simulink model "edda-ctc"  (R2021a)
settings: Solver=ode45  StartTime=0.0  StopTime=100  RelTol=1e-10
values from neighbouring files (symbols this model uses):
  g = 9.81    [alg1.m]    (also in alg2.m; edda-ctc-script.m; edda-pd-script.m)
  K0 = 1    [alg1.m]    (also in alg2.m = 10; edda-ctc-script.m = 10; edda-pd-script.m)
  K1 = 1    [alg1.m]    (also in alg2.m; edda-ctc-script.m; edda-pd-script.m)
  Theta1 = 3.1    [alg1.m]    (also in alg2.m; edda-ctc-script.m; edda-pd-script.m)
  Theta2 = 9.5    [alg1.m]    (also in alg2.m; edda-ctc-script.m; edda-pd-script.m)
  Theta3 = 0.24    [alg1.m]    (also in alg2.m; edda-ctc-script.m; edda-pd-script.m)
  Theta4 = 0.77    [alg1.m]    (also in alg2.m; edda-ctc-script.m; edda-pd-script.m)
settings Model: Creator=lajk0  LastModifiedBy=lajk0
settings DataIOCC: ReturnWorkspaceOutputs=off

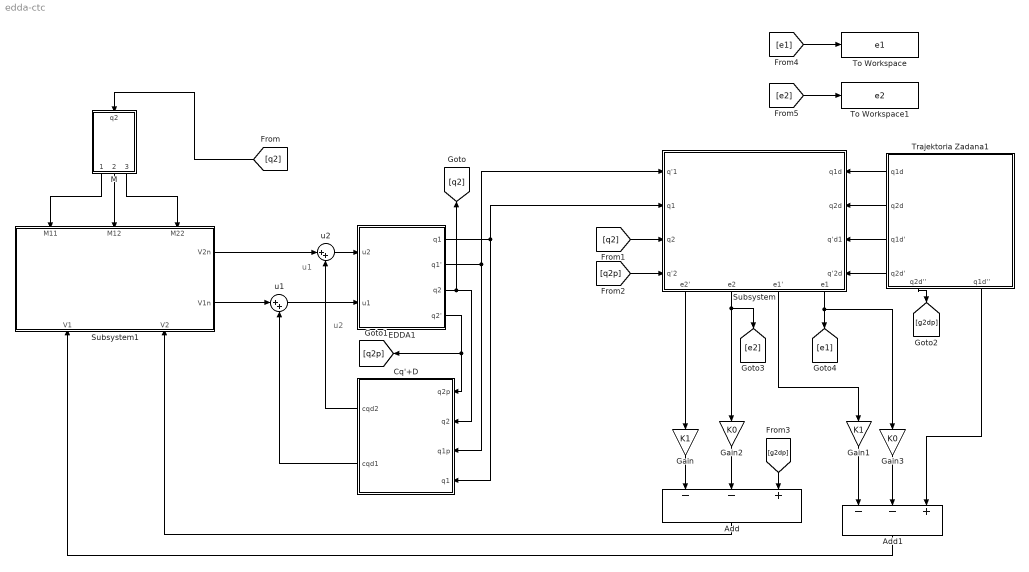
== system edda-ctc ==
  note: u1
  note: u2
  Add : Sum  Inputs=--+
  Add1 : Sum  Inputs=--+
  Cq'+D : Subsystem
  EDDA1 : Subsystem
  Gain : Gain  Gain=K1
  Gain1 : Gain  Gain=K1
  Gain2 : Gain  Gain=K0
  Gain3 : Gain  Gain=K0
  M : MATLAB Function  TreatAsAtomicUnit=on
  Subsystem : Subsystem
      settings: PortSchema="{\"entries\":[{\"content\":{\"sides\":[{\"content\":{\"connectorIds\":[\"In1\",\"In2\",\"In3\",\"In4\"]},\"type\":\"ConnectorPlacement.EquallySpacedRectSide\",\"uuid\":\"3303e5f2-67ee-45b6-97a0-23586c48cd6c\"},{\"content\":{\"connectorIds\":[\"In5\",\"In6\",\"In7\",\"In8\"],\"side\":\"RIGHT\"},\"type\":\"ConnectorPlacement.EquallySpacedRectSide\",\"uuid\":\"1b0957a8-25ba-4d38-8463-d98e460b7b4b\"},{\"content\":{\"connectorIds\":[],\"side\":\"TOP\"},\"type\":\"ConnectorPlacement.EquallySpacedRectSide\",\"uuid\":\"dcd10877-6c12-4756-8cd6-2aa2f8a0ea7e\"},{\"content\":{\"connectorIds\":[\"Out1\",\"Out2\",\"Out3\",\"Out4\"],\"side\":\"BOTTOM\"},\"type\":\"ConnectorPlacement.EquallySpacedRectSide\",\"uuid\":\"1d649839-c0ac-4460-a6a4-f4770d1aa05c\"}]},\"type\":\"ConnectorPlacement.EquallySpacedConnector\",\"uuid\":\"78f92c88-f617-45b2-819c-155b2b56e8f4\"}],\"packageUris\":[\"http://schema.mathworks.com/mf0/Connector/R2020b\"],\"version\":\"1.0\"}"
  Subsystem1 : Subsystem
      settings: PortSchema="{\"entries\":[{\"content\":{\"sides\":[{\"content\":{\"connectorIds\":[]},\"type\":\"ConnectorPlacement.EquallySpacedRectSide\",\"uuid\":\"3303e5f2-67ee-45b6-97a0-23586c48cd6c\"},{\"content\":{\"connectorIds\":[\"Out1\",\"Out2\"],\"side\":\"RIGHT\"},\"type\":\"ConnectorPlacement.EquallySpacedRectSide\",\"uuid\":\"1b0957a8-25ba-4d38-8463-d98e460b7b4b\"},{\"content\":{\"connectorIds\":[\"In1\",\"In2\",\"In3\"],\"side\":\"TOP\"},\"type\":\"ConnectorPlacement.EquallySpacedRectSide\",\"uuid\":\"dcd10877-6c12-4756-8cd6-2aa2f8a0ea7e\"},{\"content\":{\"connectorIds\":[\"In4\",\"In5\"],\"side\":\"BOTTOM\"},\"type\":\"ConnectorPlacement.EquallySpacedRectSide\",\"uuid\":\"1d649839-c0ac-4460-a6a4-f4770d1aa05c\"}]},\"type\":\"ConnectorPlacement.EquallySpacedConnector\",\"uuid\":\"78f92c88-f617-45b2-819c-155b2b56e8f4\"}],\"packageUris\":[\"http://schema.mathworks.com/mf0/Connector/R2020b\"],\"version\":\"1.0\"}"
  To Workspace : ToWorkspace  VariableName=e1  SampleTime=-1
  To Workspace1 : ToWorkspace  VariableName=e2  SampleTime=-1
  Trajektoria Zadana1 : Subsystem
      settings: PortSchema="{\"entries\":[{\"content\":{\"sides\":[{\"content\":{\"connectorIds\":[]},\"type\":\"ConnectorPlacement.EquallySpacedRectSide\",\"uuid\":\"a4d08f75-1dc7-466a-b8d3-29851c7ae152\"},{\"content\":{\"connectorIds\":[\"Out1\",\"Out2\",\"Out3\",\"Out4\"],\"side\":\"RIGHT\"},\"type\":\"ConnectorPlacement.EquallySpacedRectSide\",\"uuid\":\"ff34c384-9eaf-40f0-a095-f6b1ecae056f\"},{\"content\":{\"connectorIds\":[],\"side\":\"TOP\"},\"type\":\"ConnectorPlacement.EquallySpacedRectSide\",\"uuid\":\"6867b8fb-0822-4a57-a58b-a865865a3d34\"},{\"content\":{\"connectorIds\":[\"Out5\",\"Out6\"],\"side\":\"BOTTOM\"},\"type\":\"ConnectorPlacement.EquallySpacedRectSide\",\"uuid\":\"76455bd9-72e5-42ca-add8-84252a544d0e\"}]},\"type\":\"ConnectorPlacement.EquallySpacedConnector\",\"uuid\":\"c8ab04dd-95eb-4c57-b11e-dacd8059db0e\"}],\"packageUris\":[\"http://schema.mathworks.com/mf0/Connector/R2020b\"],\"version\":\"1.0\"}"
  u1 : Sum  Inputs=|++
  u2 : Sum  Inputs=|++
  wires:
  EDDA1/4(q2') -> Cq'+D/1(q2p), [q2p]
  EDDA1/3(q2) -> Cq'+D/2(q2), [q2]
  EDDA1/2(q1') -> Subsystem/1(q'1), Cq'+D/3(q1p)
  Cq'+D/2(cqd1) -> u1/2
  Cq'+D/1(cqd2) -> u2/2
  u1/1 -> EDDA1/2(u1)
  u2/1 -> EDDA1/1(u2)
  EDDA1/1(q1) -> Cq'+D/4(q1), Subsystem/2(q1)
  [q2] -> M/1(q2)
  Trajektoria Zadana1/1(q1d) -> Subsystem/5(q1d)
  Trajektoria Zadana1/2(q2d) -> Subsystem/6(q2d)
  Trajektoria Zadana1/3(q1d') -> Subsystem/7(q'd1)
  Trajektoria Zadana1/4(q2d') -> Subsystem/8(q'2d)
  [q2] -> Subsystem/3(q2)
  [q2p] -> Subsystem/4(q'2)
  M/1(M11) -> Subsystem1/1(M11)
  M/2(M12) -> Subsystem1/2(M12)
  M/3(M22) -> Subsystem1/3(M22)
  Subsystem1/2(V1n) -> u1/1
  Subsystem1/1(V2n) -> u2/1
  Subsystem/1(e2') -> Gain/1
  Subsystem/3(e1') -> Gain1/1
  Subsystem/2(e2) -> Gain2/1, [e2]
  Subsystem/4(e1) -> [e1], Gain3/1
  Trajektoria Zadana1/5(q1d'') -> Add1/3
  Gain/1 -> Add/1
  Gain2/1 -> Add/2
  Gain1/1 -> Add1/1
  Gain3/1 -> Add1/2
  Add/1 -> Subsystem1/5(V2)
  Add1/1 -> Subsystem1/4(V1)
  Trajektoria Zadana1/6(q2d'') -> [g2dp]
  [g2dp] -> Add/3
  [e2] -> To Workspace1/1
  [e1] -> To Workspace/1

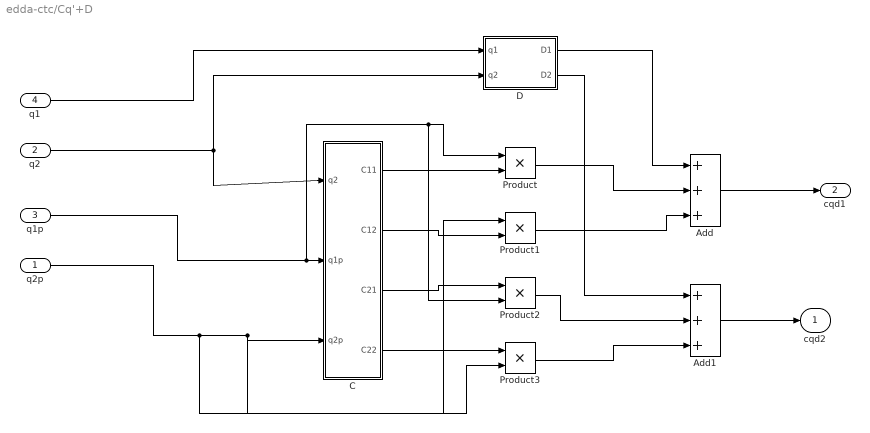
== system edda-ctc/Cq'+D ==
  q2p : Inport
  q2 : Inport  Port=2
  q1p : Inport  Port=3
  q1 : Inport  Port=4
  Add : Sum  Inputs=+++
  Add1 : Sum  Inputs=+++
  C : MATLAB Function  TreatAsAtomicUnit=on
  D : MATLAB Function  TreatAsAtomicUnit=on
  Product{,1..3} (4 alike) : Product
  cqd2 : Outport
  cqd1 : Outport  Port=2
  wires:
  q2/1 -> D/2(q2), C/1(q2)
  q1/1 -> D/1(q1)
  q2p/1 -> Product3/2, Product1/1, C/3(q2p)
  q1p/1 -> Product2/2, Product/1, C/2(q1p)
  C/1(C11) -> Product/2
  C/2(C12) -> Product1/2
  C/3(C21) -> Product2/1
  C/4(C22) -> Product3/1
  Product/1 -> Add/2
  Product1/1 -> Add/3
  D/1(D1) -> Add/1
  D/2(D2) -> Add1/1
  Product2/1 -> Add1/2
  Product3/1 -> Add1/3
  Add/1 -> cqd1/1
  Add1/1 -> cqd2/1

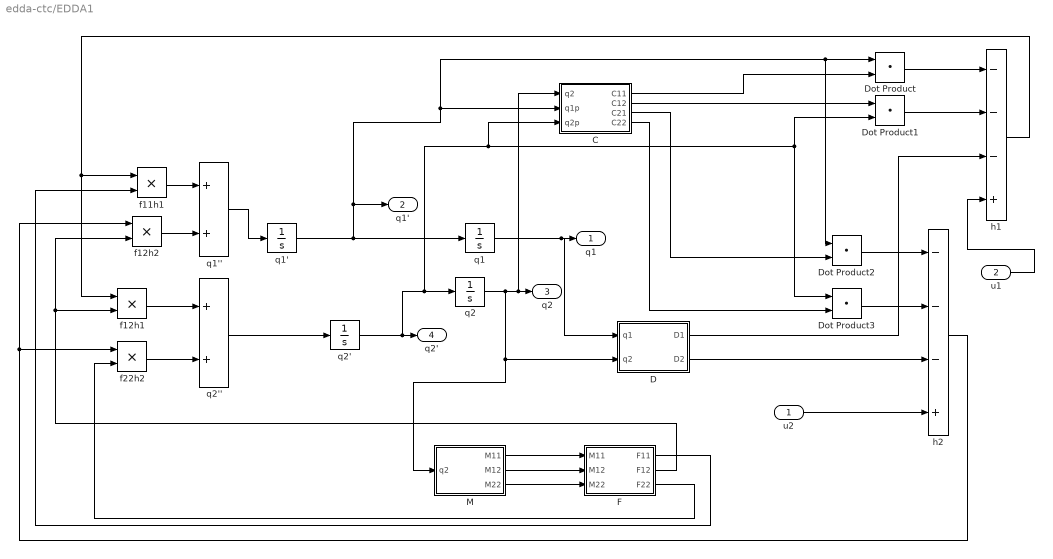
== system edda-ctc/EDDA1 ==
  u2 : Inport
  u1 : Inport  Port=2
  " q1" : Integrator
  " q1'" : Integrator
  " q2" : Integrator
  " q2'" : Integrator
  C : MATLAB Function  TreatAsAtomicUnit=on
  D : MATLAB Function  TreatAsAtomicUnit=on
  Dot Product{,1..3} (4 alike) : DotProduct  InputSameDT=on  OutDataTypeStr=Inherit: Inherit via internal rule
  F : MATLAB Function  TreatAsAtomicUnit=on
  M : MATLAB Function  TreatAsAtomicUnit=on
  f11h1 : Product
  f12h1 : Product
  f12h2 : Product
  f22h2 : Product
  h1 : Sum  Inputs=---+
  h2 : Sum  Inputs=---+
  q1'' : Sum
  q2'' : Sum
  q1 : Outport
  q1' : Outport  Port=2
  q2 : Outport  Port=3
  q2' : Outport  Port=4
  wires:
  u1/1 -> h1/4
  u2/1 -> h2/4
  " q2'"/1 -> C/3(q2p), Dot Product3/1, Dot Product1/2, " q2"/1, q2'/1
  " q2"/1 -> M/1(q2), D/2(q2), q2/1, C/1(q2)
  " q1"/1 -> D/1(q1), q1/1
  M/1(M11) -> F/1(M11)
  M/2(M12) -> F/2(M12)
  M/3(M22) -> F/3(M22)
  Dot Product/1 -> h1/1
  C/1(C11) -> Dot Product/2
  Dot Product1/1 -> h1/2
  C/2(C12) -> Dot Product1/1
  D/1(D1) -> h1/3
  D/2(D2) -> h2/3
  Dot Product2/1 -> h2/1
  Dot Product3/1 -> h2/2
  C/3(C21) -> Dot Product2/2
  C/4(C22) -> Dot Product3/2
  " q1'"/1 -> q1'/1, Dot Product2/1, Dot Product/1, C/2(q1p), " q1"/1
  h1/1 -> f12h1/1, f11h1/1
  F/3(F22) -> f22h2/2
  F/2(F12) -> f12h2/2, f12h1/2
  F/1(F11) -> f11h1/2
  q1''/1 -> " q1'"/1
  q2''/1 -> " q2'"/1
  f11h1/1 -> q1''/1
  f12h2/1 -> q1''/2
  f12h1/1 -> q2''/1
  f22h2/1 -> q2''/2
  h2/1 -> f12h2/1, f22h2/1

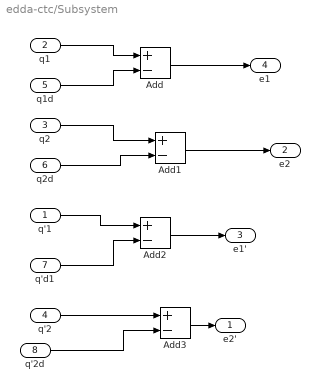
== system edda-ctc/Subsystem ==
  q'1 : Inport
  q1 : Inport  Port=2
  q2 : Inport  Port=3
  q'2 : Inport  Port=4
  q1d : Inport  Port=5
  q2d : Inport  Port=6
  q'd1 : Inport  Port=7
  q'2d : Inport  Port=8
  Add{,1..3} (4 alike) : Sum  Inputs=+-
  e2' : Outport
  e2 : Outport  Port=2
  e1' : Outport  Port=3
  e1 : Outport  Port=4
  wires:
  q1/1 -> Add/1
  q2/1 -> Add1/1
  q'2/1 -> Add3/1
  q1d/1 -> Add/2
  q2d/1 -> Add1/2
  q'1/1 -> Add2/1
  q'd1/1 -> Add2/2
  Add1/1 -> e2/1
  Add/1 -> e1/1
  Add2/1 -> e1'/1
  Add3/1 -> e2'/1
  q'2d/1 -> Add3/2

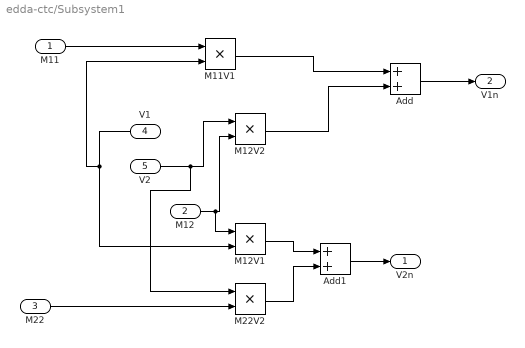
== system edda-ctc/Subsystem1 ==
  M11 : Inport
  M12 : Inport  Port=2
  M22 : Inport  Port=3
  V1 : Inport  Port=4
  V2 : Inport  Port=5
  Add : Sum
  Add1 : Sum
  M11V1 : Product
  M12V1 : Product
  M12V2 : Product
  M22V2 : Product
  V2n : Outport
  V1n : Outport  Port=2
  wires:
  M11/1 -> M11V1/1
  M22/1 -> M22V2/2
  M12/1 -> M12V1/1, M12V2/2
  Add/1 -> V1n/1
  Add1/1 -> V2n/1
  V2/1 -> M12V2/1, M22V2/1
  V1/1 -> M12V1/2, M11V1/2
  M11V1/1 -> Add/1
  M12V2/1 -> Add/2
  M12V1/1 -> Add1/1
  M22V2/1 -> Add1/2

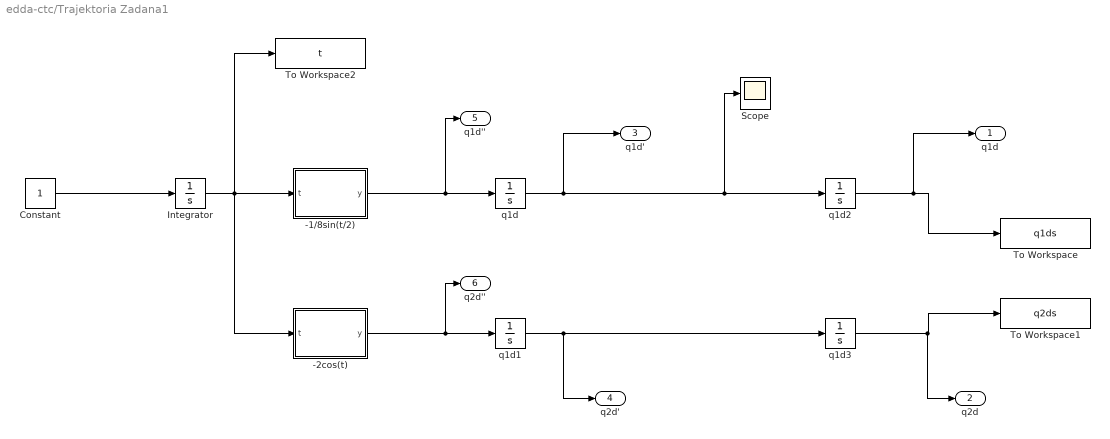
== system edda-ctc/Trajektoria Zadana1 ==
  " q1d" : Integrator  InitialCondition=1/4
  " q1d1" : Integrator
  " q1d2" : Integrator
  " q1d3" : Integrator  InitialCondition=2
  -1/8sin(t/2) : MATLAB Function  TreatAsAtomicUnit=on
  -2cos(t) : MATLAB Function  TreatAsAtomicUnit=on
  Constant : Constant
  Integrator : Integrator
  Scope : Scope
  To Workspace : ToWorkspace  VariableName=q1ds  SampleTime=-1
  To Workspace1 : ToWorkspace  VariableName=q2ds  SampleTime=-1
  To Workspace2 : ToWorkspace  VariableName=t  SampleTime=-1
  q1d : Outport
  q2d : Outport  Port=2
  q1d' : Outport  Port=3
  q2d' : Outport  Port=4
  q1d'' : Outport  Port=5
  q2d'' : Outport  Port=6
  wires:
  Integrator/1 -> To Workspace2/1, -2cos(t)/1(t), -1/8sin(t/2)/1(t)
  -1/8sin(t/2)/1(y) -> q1d''/1, " q1d"/1
  " q1d"/1 -> Scope/1, " q1d2"/1, q1d'/1
  -2cos(t)/1(y) -> q2d''/1, " q1d1"/1
  " q1d1"/1 -> " q1d3"/1, q2d'/1
  Constant/1 -> Integrator/1
  " q1d2"/1 -> q1d/1, To Workspace/1
  " q1d3"/1 -> q2d/1, To Workspace1/1

== matlab function edda-ctc/M ==
  data: q2 input; M11 output; M12 output; M22 output; Theta1 parameter; Theta3 parameter; Theta4 parameter
function [M11, M12,  M22]= fcn(q2, Theta1,  Theta3, Theta4)

M11=Theta1+0.6*Theta4*cos(q2);
M12=Theta3+0.3*Theta4*cos(q2);
%M21=Theta3+0.3*Theta4*cos(q2);
M22=Theta3;

== matlab function edda-ctc/EDDA1/C ==
  data: q2 input; C11 output; q1p input; q2p input; C12 output; C21 output; C22 output; Theta4 parameter
function [C11,C12,C21,C22]= fcn(q2 ,q1p  ,q2p, Theta4)
a=0.3*Theta4*sin(q2);
C11=-q2p*a;
C12=-(q1p+q2p)*a;
C21=q1p*a;
C22=0*a;

== matlab function edda-ctc/EDDA1/D ==
  data: q1 input; D1 output; q2 input; D2 output; g parameter; Theta4 parameter; Theta2 parameter
function [D1, D2]= fcn(q1, q2, g, Theta4, Theta2)

D1=Theta2*cos(q1)+Theta4*cos(q1+q2)*g;
D2=Theta4*cos(q1+q2)*g;

== matlab function edda-ctc/EDDA1/F ==
  data: M11 input; F11 output; M12 input; M22 input; F12 output; F22 output
function [F11, F12,  F22]= fcn(M11, M12,  M22)

Det=M11*M22-M12*M12;
F11=M22/Det;
F12=-M12/Det;
F22=M11/Det;

== matlab function edda-ctc/EDDA1/M ==
  data: q2 input; M11 output; M12 output; M22 output; Theta1 parameter; Theta3 parameter; Theta4 parameter
function [M11, M12,  M22]= fcn(q2, Theta1,  Theta3, Theta4)

M11=Theta1+0.6*Theta4*cos(q2);
M12=Theta3+0.3*Theta4*cos(q2);
%M21=Theta3+0.3*Theta4*cos(q2);
M22=Theta3;

== matlab function edda-ctc/Trajektoria Zadana1/-2cos(t) ==
  data: t input; y output
function y = fcn(t)

y = -2*cos(t);

== matlab function edda-ctc/Trajektoria Zadana1/-1//8sin(t//2) ==
  data: t input; y output
function y = fcn(t)

y =-(1/8)*sin(t/2);

== matlab function edda-ctc/Cq'+D/D ==
  data: q1 input; D1 output; q2 input; D2 output; g parameter; Theta4 parameter; Theta2 parameter
function [D1, D2]= fcn(q1, q2, g, Theta4, Theta2)

D1=Theta2*cos(q1)+Theta4*cos(q1+q2)*g;
D2=Theta4*cos(q1+q2)*g;

== matlab function edda-ctc/Cq'+D/C ==
  data: q2 input; C11 output; q1p input; q2p input; C12 output; C21 output; C22 output; Theta4 parameter
function [C11,C12,C21,C22]= fcn(q2 ,q1p  ,q2p, Theta4)
a=0.3*Theta4*sin(q2);
C11=-q2p*a;
C12=-(q1p+q2p)*a;
C21=q1p*a;
C22=0*a;
